simulink model "Mode_plus_Heading"  (R2015a)
settings: Solver=ode45  StartTime=0.0  StopTime=10.0  RelTol=1e-3
libraries: simulink x11, discretizing x1
settings Model: Creator=teme  LastModifiedBy=teme

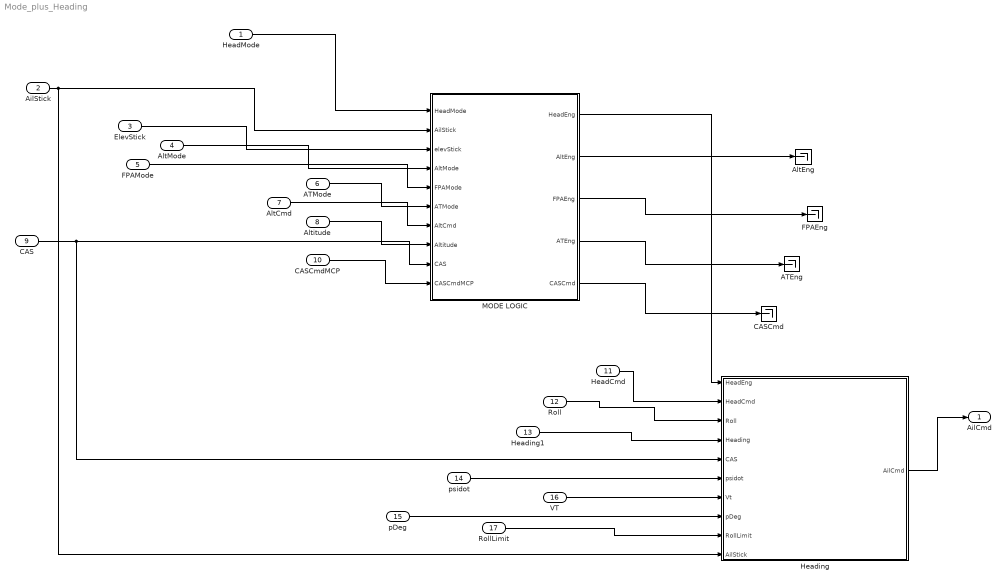
== system Mode_plus_Heading ==
  HeadMode : Inport
  AilStick : Inport  Port=2
  ElevStick : Inport  Port=3
  AltMode : Inport  Port=4
  FPAMode : Inport  Port=5
  ATMode : Inport  Port=6
  AltCmd : Inport  Port=7
  Altitude : Inport  Port=8
  CAS : Inport  Port=9
  CASCmdMCP : Inport  Port=10
  HeadCmd : Inport  Port=11
  "Roll " : Inport  Port=12
  Heading1 : Inport  Port=13
  psidot : Inport  Port=14
  pDeg : Inport  Port=15
  VT : Inport  Port=16
  RollLimit : Inport  Port=17
  ATEng : Terminator
  AltEng : Terminator
  CASCmd : Terminator
  FPAEng : Terminator
  Heading : Subsystem  TreatAsAtomicUnit=on
  MODE LOGIC : Subsystem  TreatAsAtomicUnit=on
  AilCmd : Outport
  wires:
  HeadMode/1 -> MODE LOGIC/1(HeadMode)
  AilStick/1 -> Heading/10(AilStick), MODE LOGIC/2(AilStick)
  AltMode/1 -> MODE LOGIC/4(AltMode)
  FPAMode/1 -> MODE LOGIC/5(FPAMode)
  ATMode/1 -> MODE LOGIC/6(ATMode)
  CASCmdMCP/1 -> MODE LOGIC/10(CASCmdMCP)
  MODE LOGIC/1(HeadEng) -> Heading/1(HeadEng)
  CAS/1 -> Heading/5(CAS), MODE LOGIC/9(CAS)
  AltCmd/1 -> MODE LOGIC/7(AltCmd)
  Altitude/1 -> MODE LOGIC/8(Altitude)
  ElevStick/1 -> MODE LOGIC/3(elevStick)
  Heading/1(AilCmd) -> AilCmd/1
  HeadCmd/1 -> Heading/2(HeadCmd)
  "Roll "/1 -> Heading/3(Roll)
  Heading1/1 -> Heading/4(Heading)
  psidot/1 -> Heading/6(psidot)
  pDeg/1 -> Heading/8(pDeg)
  VT/1 -> Heading/7(Vt)
  RollLimit/1 -> Heading/9(RollLimit)
  MODE LOGIC/2(AltEng) -> AltEng/1
  MODE LOGIC/3(FPAEng) -> FPAEng/1
  MODE LOGIC/4(ATEng) -> ATEng/1
  MODE LOGIC/5(CASCmd) -> CASCmd/1

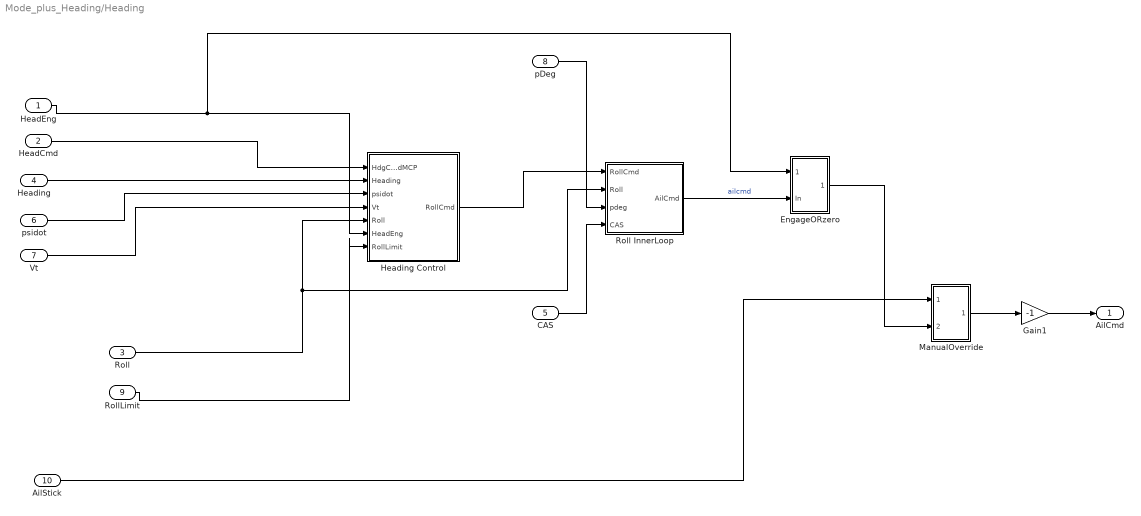
== system Mode_plus_Heading/Heading ==
  HeadEng : Inport
  HeadCmd : Inport  Port=2
  Roll : Inport  Port=3
  Heading : Inport  Port=4
  CAS : Inport  Port=5
  psidot : Inport  Port=6
  Vt : Inport  Port=7
  pDeg : Inport  Port=8
  RollLimit : Inport  Port=9
  AilStick : Inport  Port=10
  EngageORzero : Subsystem
  Gain1 : Gain  RequirementInfo={} %GIDa_6d55ac65_202a_4981_a4f5_213afcb30605  Gain=-1  SaturateOnIntegerOverflow=on  OutDataTypeStr=Inherit: Same as input  ParamDataTypeStr=Inherit: Same as input
  Heading Control : Subsystem  RequirementInfo={'other' '..\..\tcm_requirements.docx' '@Simulink_requirement_item_16' 'true' 'Heading Control' '' } %GIDa_029c738f_f50b_45d2_a289_cf2e96dbaa78  TreatAsAtomicUnit=on
  ManualOverride : Subsystem
  Roll InnerLoop : Subsystem  RequirementInfo={'other' '..\..\tcm_requirements.docx' '@Simulink_requirement_item_18' 'true' 'Roll InnerLoop' '' } %GIDa_cbfef998_9b02_4a35_a4cd_5451b3fb610d  TreatAsAtomicUnit=on
  AilCmd : Outport
  wires:
  pDeg/1 -> Roll InnerLoop/3(pdeg)
  Vt/1 -> Heading Control/4(Vt)
  psidot/1 -> Heading Control/3(psidot)
  Heading/1 -> Heading Control/2(Heading)
  Roll/1 -> Heading Control/5(Roll), Roll InnerLoop/2(Roll)
  Heading Control/1(RollCmd) -> Roll InnerLoop/1(RollCmd)
  Roll InnerLoop/1(AilCmd) -> EngageORzero/2(In)  "ailcmd"
  HeadCmd/1 -> Heading Control/1(HdgCmdMCP)
  HeadEng/1 -> EngageORzero/1(Engage), Heading Control/6(HeadEng)
  CAS/1 -> Roll InnerLoop/4(CAS)
  RollLimit/1 -> Heading Control/7(RollLimit)
  ManualOverride/1(Out) -> Gain1/1
  AilStick/1 -> ManualOverride/1(Man)
  Gain1/1 -> AilCmd/1
  EngageORzero/1(Out) -> ManualOverride/2(Auto)

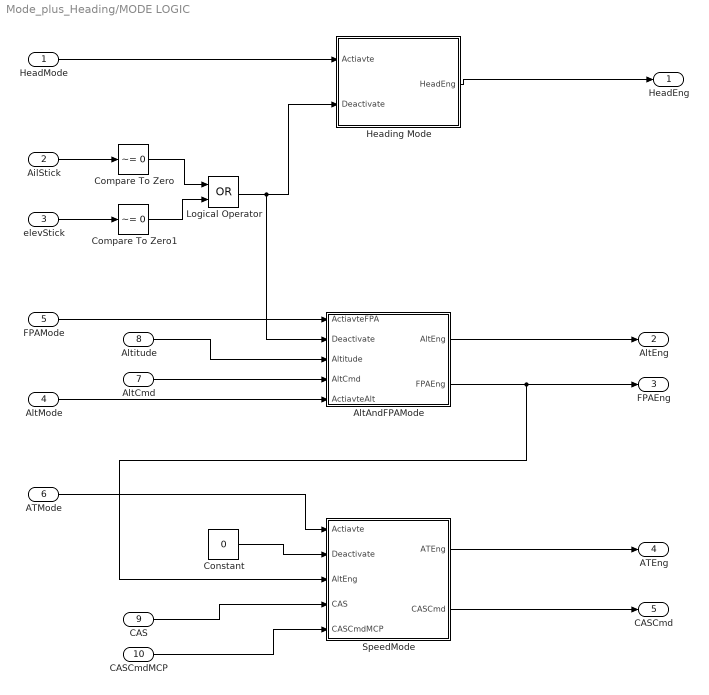
== system Mode_plus_Heading/MODE LOGIC ==
  HeadMode : Inport
  AilStick : Inport  Port=2
  elevStick : Inport  Port=3
  AltMode : Inport  Port=4
  FPAMode : Inport  Port=5
  ATMode : Inport  Port=6
  AltCmd : Inport  Port=7
  Altitude : Inport  Port=8
  CAS : Inport  Port=9
  CASCmdMCP : Inport  Port=10
  AltAndFPAMode : Subsystem  TreatAsAtomicUnit=on
  Compare To Zero : simulink/Logic and Bit Operations/Compare To Zero  relop=~=  OutDataTypeStr=boolean
  Compare To Zero1 : simulink/Logic and Bit Operations/Compare To Zero  relop=~=  OutDataTypeStr=boolean
  Constant : Constant  Value=0
  Heading Mode : Subsystem  TreatAsAtomicUnit=on
  Logical Operator : Logic  Operator=OR  AllPortsSameDT=off  OutDataTypeStr=boolean
  SpeedMode : Subsystem  TreatAsAtomicUnit=on
  HeadEng : Outport
  AltEng : Outport  Port=2
  FPAEng : Outport  Port=3
  ATEng : Outport  Port=4
  CASCmd : Outport  Port=5
  wires:
  SpeedMode/1(ATEng) -> ATEng/1
  AilStick/1 -> Compare To Zero/1
  Constant/1 -> SpeedMode/2(Deactivate)
  AltAndFPAMode/2(FPAEng) -> FPAEng/1, SpeedMode/3(AltEng)
  AltAndFPAMode/1(AltEng) -> AltEng/1
  Heading Mode/1(HeadEng) -> HeadEng/1
  HeadMode/1 -> Heading Mode/1(Actiavte)
  Compare To Zero1/1 -> Logical Operator/2
  Compare To Zero/1 -> Logical Operator/1
  elevStick/1 -> Compare To Zero1/1
  ATMode/1 -> SpeedMode/1(Actiavte)
  FPAMode/1 -> AltAndFPAMode/1(ActiavteFPA)
  Altitude/1 -> AltAndFPAMode/3(Altitude)
  AltMode/1 -> AltAndFPAMode/5(ActiavteAlt)
  Logical Operator/1 -> AltAndFPAMode/2(Deactivate), Heading Mode/2(Deactivate)
  CASCmdMCP/1 -> SpeedMode/5(CASCmdMCP)
  AltCmd/1 -> AltAndFPAMode/4(AltCmd)
  SpeedMode/2(CASCmd) -> CASCmd/1
  CAS/1 -> SpeedMode/4(CAS)

== system Mode_plus_Heading/Heading/EngageORzero ==
  Engage : Inport
  In : Inport  Port=2
  Logical Operator5 : Logic  RequirementInfo={} %GIDa_6b22acc9_652a_4444_ba60_66174211b3d7  AllPortsSameDT=off  OutDataTypeStr=boolean
  Switch1 : Switch  RequirementInfo={} %GIDa_a25acb75_51aa_42d7_a9cb_36d9cbb78c82  Threshold=0.5
  zero10 : Constant  RequirementInfo={} %GIDa_53b8c13b_6898_41e6_9738_617635f10221
  zero9 : Constant  RequirementInfo={} %GIDa_0f665773_e07d_469a_a003_01a4a005c292  Value=0
  Out : Outport
  wires:
  Engage/1 -> Logical Operator5/1
  zero10/1 -> Logical Operator5/2
  zero9/1 -> Switch1/3
  In/1 -> Switch1/1
  Logical Operator5/1 -> Switch1/2
  Switch1/1 -> Out/1

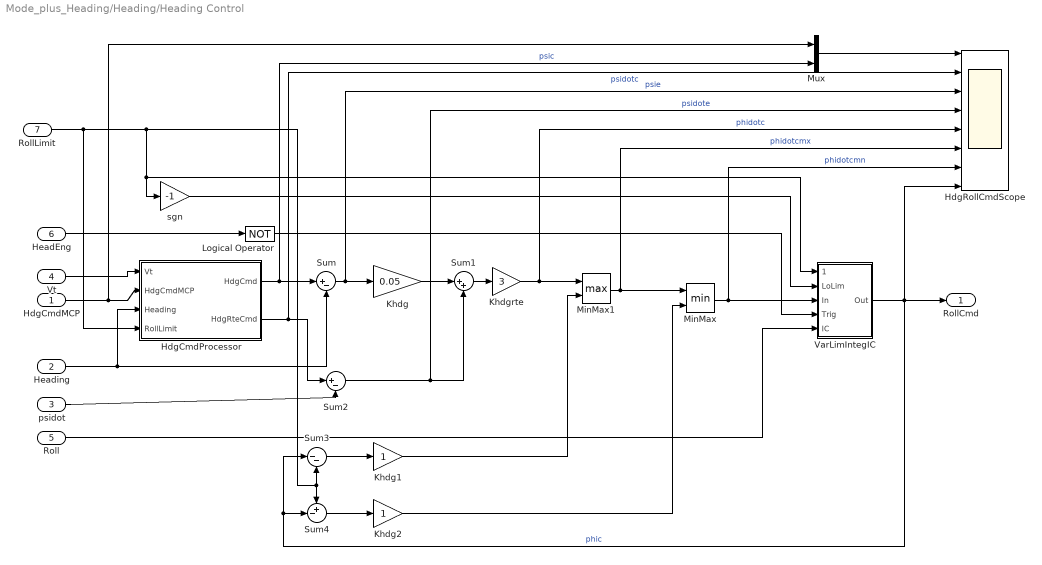
== system Mode_plus_Heading/Heading/Heading Control ==
  HdgCmdMCP : Inport  RequirementInfo={} %GIDa_1cca2c5c_8ee7_4499_91b8_56e2b6de226b
  Heading : Inport  RequirementInfo={} %GIDa_335b309e_b3fa_45a8_b4d1_17ef1ad18bf7  Port=2
  psidot : Inport  RequirementInfo={} %GIDa_0ad6fda9_8653_402a_9e5f_aea66e3ef369  Port=3
  Vt : Inport  RequirementInfo={} %GIDa_f5693dda_631a_4bfe_baea_8b34b02d8022  Port=4
  Roll : Inport  RequirementInfo={} %GIDa_593befd8_2743_476a_a356_0063a557a98d  Port=5
  HeadEng : Inport  RequirementInfo={} %GIDa_e8b59cf9_df4b_4ada_848e_4da61a3fd8b6  Port=6
  RollLimit : Inport  Port=7
  HdgCmdProcessor : Subsystem  RequirementInfo={} %GIDa_26e06564_c060_46ec_be4a_5847d57d6a81
  HdgRollCmdScope : Scope  NumInputPorts=8
      settings: RequirementInfo={} %GIDa_862353d9_0e7c_4d5b_85e1_9c9746c3fb38  YMin=-30~-30~-10~-10~-4~-10~0~-5  YMax=30~30~10~10~4~10~1~5  SaveName=ScopeData7
  Khdg : Gain  RequirementInfo={} %GIDa_c081e4bf_f383_4484_b7bd_3abc2cab8bec  Gain=0.05
  Khdg1 : Gain  RequirementInfo={} %GIDa_08836d3b_c1d7_4517_b088_b37e47d972bd
  Khdg2 : Gain  RequirementInfo={} %GIDa_3aec3149_958f_47ac_94ee_3d28a77fc3f5
  Khdgrte : Gain  RequirementInfo={} %GIDa_53d347bb_462f_4886_bdb2_badb643f02f4  Gain=3
  Logical Operator : Logic  RequirementInfo={} %GIDa_4b58cabb_2297_487d_8b60_ff4175741a78  Operator=NOT  AllPortsSameDT=off  OutDataTypeStr=boolean
  MinMax : MinMax  RequirementInfo={} %GIDa_e41d7ecf_e4e1_4710_b8b1_1fc040f0e9f7  Inputs=2
  MinMax1 : MinMax  RequirementInfo={} %GIDa_a4542adf_d925_494d_a294_9fe772a2ae1b  Function=max  Inputs=2
  Mux : Mux  RequirementInfo={} %GIDa_470c3405_5717_4020_8437_1a783ba94da4  Inputs=2
  Sum : Sum  RequirementInfo={} %GIDa_6c1efd1c_9252_4e5c_91dd_39c700892261  Inputs=|+-
  Sum1 : Sum  RequirementInfo={} %GIDa_6cd8dae3_1c4e_4eaf_8404_21dd295850e0  Inputs=|++
  Sum2 : Sum  RequirementInfo={} %GIDa_9d15b97d_5642_4675_a5ca_204c66429b4e  Inputs=|+-
  Sum3 : Sum  RequirementInfo={} %GIDa_2fe000b9_a62e_4a0f_869a_3cd4af55113b  Inputs=|--
  Sum4 : Sum  RequirementInfo={} %GIDa_c46e2e29_3542_4ab2_a31d_585bcdcc8614  Inputs=+-|
  VarLimIntegIC : Subsystem  RequirementInfo={} %GIDa_71edeeee_c821_4f10_9933_03fc141b3c8d
  sgn : Gain  RequirementInfo={} %GIDa_f2aeabed_4671_4607_b0d8_c27b93e0bf37  Gain=-1
  RollCmd : Outport  RequirementInfo={} %GIDa_4ce52d3c_e4b9_4db6_a642_099518279411
  wires:
  Heading/1 -> Sum/2, HdgCmdProcessor/3(Heading)
  HdgCmdProcessor/1(HdgCmd) -> Sum/1, Mux/2  "psic"
  Sum/1 -> Khdg/1, HdgRollCmdScope/3  "psie"
  Khdg/1 -> Sum1/1
  Sum2/1 -> Sum1/2, HdgRollCmdScope/4  "psidote"
  HdgCmdProcessor/2(HdgRteCmd) -> Sum2/1, HdgRollCmdScope/2  "psidotc"
  psidot/1 -> Sum2/2
  Vt/1 -> HdgCmdProcessor/1(Vt)
  HdgCmdMCP/1 -> HdgCmdProcessor/2(HdgCmdMCP), Mux/1
  VarLimIntegIC/1(Out) -> RollCmd/1, Sum3/1, Sum4/2, HdgRollCmdScope/8  "phic"
  RollLimit/1 -> HdgCmdProcessor/4(RollLimit), Sum4/1, Sum3/2, VarLimIntegIC/1(UpLim), sgn/1
  sgn/1 -> VarLimIntegIC/2(LoLim)
  Sum1/1 -> Khdgrte/1
  MinMax1/1 -> MinMax/1, HdgRollCmdScope/6  "phidotcmx"
  MinMax/1 -> VarLimIntegIC/3(In), HdgRollCmdScope/7  "phidotcmn"
  HeadEng/1 -> Logical Operator/1
  Sum3/1 -> Khdg1/1
  Sum4/1 -> Khdg2/1
  Khdg1/1 -> MinMax1/2
  Khdg2/1 -> MinMax/2
  Roll/1 -> VarLimIntegIC/5(IC)
  Khdgrte/1 -> MinMax1/1, HdgRollCmdScope/5  "phidotc"
  Logical Operator/1 -> VarLimIntegIC/4(Trig)
  Mux/1 -> HdgRollCmdScope/1

== system Mode_plus_Heading/Heading/ManualOverride ==
  Man : Inport
  Auto : Inport  Port=2
  Switch1 : Switch  RequirementInfo={} %GIDa_e9c946ef_c3db_4bff_aed9_ae767ef4d81f  Criteria=u2 ~= 0  Threshold=0.5
  Out : Outport
  wires:
  Man/1 -> Switch1/3, Switch1/2
  Auto/1 -> Switch1/1
  Switch1/1 -> Out/1

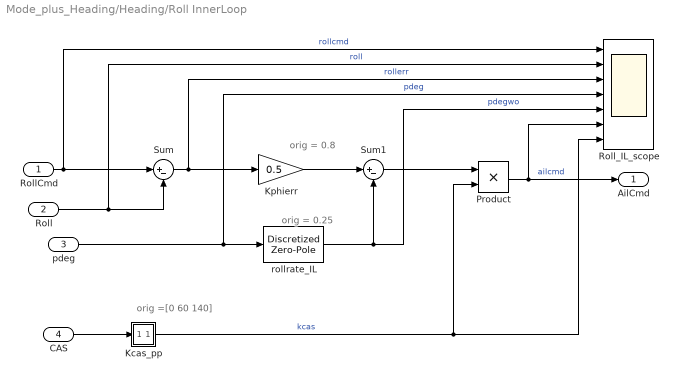
== system Mode_plus_Heading/Heading/Roll InnerLoop ==
  note: orig =[0 60 140]
  note: orig = 0.25
  note: orig = 0.8
  RollCmd : Inport  RequirementInfo={} %GIDa_d025a660_cca0_4be3_be06_f9a4dfc86269
  Roll : Inport  RequirementInfo={} %GIDa_e417ba20_aa70_4b95_9916_e8dd209e2685  Port=2
  pdeg : Inport  RequirementInfo={} %GIDa_36f75b87_1287_4d91_9dd1_6a1f7713c617  Port=3
  CAS : Inport  RequirementInfo={} %GIDa_f5e5b1c2_d48b_4547_abd4_42af90480919  Port=4
  Kcas_pp : Subsystem  TreatAsAtomicUnit=on
  Kphierr : Gain  RequirementInfo={} %GIDa_4a49e338_8293_4eab_bd1b_6b3b87e03ed9  Gain=0.5
  Product : Product  RequirementInfo={} %GIDa_b6bb309d_f019_4adc_b849_d0e1434187e8  RndMeth=Zero
  Roll_IL_scope : Scope  NumInputPorts=7
      settings: RequirementInfo={} %GIDa_cdfba529_0977_4006_adbd_37c3f846a021  YMin=-30~-30~-10~-10~-4~-10~0  YMax=30~30~10~10~4~10~1  SaveName=ScopeData5
  Sum : Sum  RequirementInfo={} %GIDa_8570fcab_2296_4031_bbbc_4321a9111662  Inputs=|+-
  Sum1 : Sum  RequirementInfo={} %GIDa_b2216589_c422_4707_aad7_b64095d3debb  Inputs=|+-
  rollrate_IL : discretizing/Discretized Zero-Pole  RequirementInfo={} %GIDa_636569be_bc7e_4244_84a4_4a62b7fc0808  Zeros=0  Poles=-0.5  Gain=0.00645  AbsTol=auto  SampleTime=1.0  method=zoh  Wc=1
  AilCmd : Outport  RequirementInfo={} %GIDa_5926b7f8_9769_4f97_a0ed_432ffd436784
  wires:
  Product/1 -> AilCmd/1, Roll_IL_scope/6  "ailcmd"
  Kcas_pp/1(Out) -> Product/2, Roll_IL_scope/7  "kcas"
  Sum1/1 -> Product/1
  CAS/1 -> Kcas_pp/1(In)
  rollrate_IL/1 -> Sum1/2, Roll_IL_scope/5  "pdegwo"
  pdeg/1 -> rollrate_IL/1, Roll_IL_scope/4  "pdeg"
  Kphierr/1 -> Sum1/1
  Roll/1 -> Sum/2, Roll_IL_scope/2  "roll"
  Sum/1 -> Kphierr/1, Roll_IL_scope/3  "rollerr"
  RollCmd/1 -> Sum/1, Roll_IL_scope/1  "rollcmd"

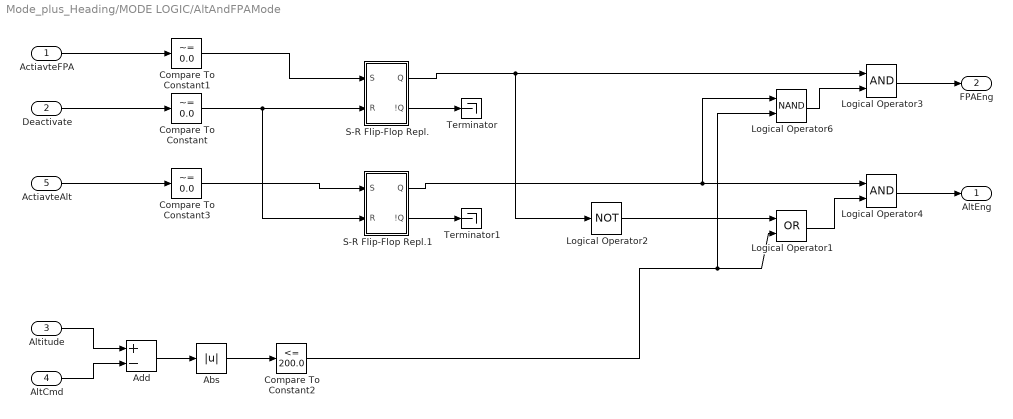
== system Mode_plus_Heading/MODE LOGIC/AltAndFPAMode ==
  ActiavteFPA : Inport
  Deactivate : Inport  Port=2
  Altitude : Inport  Port=3
  AltCmd : Inport  Port=4
  ActiavteAlt : Inport  Port=5
  Abs : Abs
  Add : Sum  Inputs=+-
  Compare To Constant : simulink/Logic and Bit Operations/Compare To Constant  relop=~=  const=0.0  OutDataTypeStr=boolean
  Compare To Constant1 : simulink/Logic and Bit Operations/Compare To Constant  relop=~=  const=0.0  OutDataTypeStr=boolean
  Compare To Constant2 : simulink/Logic and Bit Operations/Compare To Constant  relop=<=  const=200.0  OutDataTypeStr=boolean
  Compare To Constant3 : simulink/Logic and Bit Operations/Compare To Constant  relop=~=  const=0.0  OutDataTypeStr=boolean
  Logical Operator1 : Logic  Operator=OR  AllPortsSameDT=off  OutDataTypeStr=boolean
  Logical Operator2 : Logic  Operator=NOT  AllPortsSameDT=off  OutDataTypeStr=boolean
  Logical Operator3 : Logic  AllPortsSameDT=off  OutDataTypeStr=boolean
  Logical Operator4 : Logic  AllPortsSameDT=off  OutDataTypeStr=boolean
  Logical Operator6 : Logic  Operator=NAND  AllPortsSameDT=off  OutDataTypeStr=boolean
  S-R Flip-Flop Repl. : Subsystem
  S-R Flip-Flop Repl.1 : Subsystem
  Terminator : Terminator
  Terminator1 : Terminator
  AltEng : Outport
  FPAEng : Outport  Port=2
  wires:
  S-R Flip-Flop Repl./2(!Q) -> Terminator/1
  ActiavteFPA/1 -> Compare To Constant1/1
  S-R Flip-Flop Repl./1(Q) -> Logical Operator3/1, Logical Operator2/1
  Deactivate/1 -> Compare To Constant/1
  Compare To Constant1/1 -> S-R Flip-Flop Repl./1(S)
  S-R Flip-Flop Repl.1/2(!Q) -> Terminator1/1
  S-R Flip-Flop Repl.1/1(Q) -> Logical Operator6/1, Logical Operator4/1
  Compare To Constant3/1 -> S-R Flip-Flop Repl.1/1(S)
  Compare To Constant/1 -> S-R Flip-Flop Repl.1/2(R), S-R Flip-Flop Repl./2(R)
  ActiavteAlt/1 -> Compare To Constant3/1
  Altitude/1 -> Add/1
  AltCmd/1 -> Add/2
  Add/1 -> Abs/1
  Abs/1 -> Compare To Constant2/1
  Logical Operator3/1 -> FPAEng/1
  Logical Operator2/1 -> Logical Operator1/1
  Logical Operator4/1 -> AltEng/1
  Compare To Constant2/1 -> Logical Operator6/2, Logical Operator1/2
  Logical Operator1/1 -> Logical Operator4/2
  Logical Operator6/1 -> Logical Operator3/2

== system Mode_plus_Heading/MODE LOGIC/Heading Mode ==
  Actiavte : Inport
  Deactivate : Inport  Port=2
  Compare To Constant : simulink/Logic and Bit Operations/Compare To Constant  relop=~=  const=0.0  OutDataTypeStr=boolean
  Compare To Constant1 : simulink/Logic and Bit Operations/Compare To Constant  relop=~=  const=0.0  OutDataTypeStr=boolean
  S-R Flip-Flop Repl. : Subsystem
  Terminator : Terminator
  HeadEng : Outport
  wires:
  S-R Flip-Flop Repl./2(!Q) -> Terminator/1
  Actiavte/1 -> Compare To Constant1/1
  S-R Flip-Flop Repl./1(Q) -> HeadEng/1
  Deactivate/1 -> Compare To Constant/1
  Compare To Constant1/1 -> S-R Flip-Flop Repl./1(S)
  Compare To Constant/1 -> S-R Flip-Flop Repl./2(R)

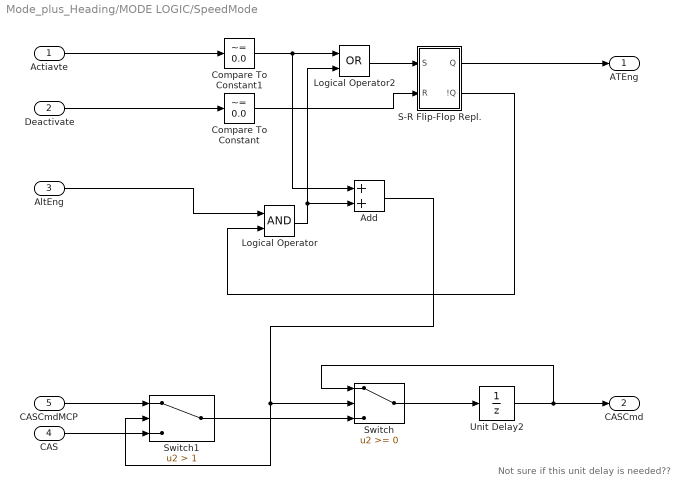
== system Mode_plus_Heading/MODE LOGIC/SpeedMode ==
  note: Not sure if this unit delay is needed??
  Actiavte : Inport
  Deactivate : Inport  Port=2
  AltEng : Inport  Port=3
  CAS : Inport  Port=4
  CASCmdMCP : Inport  Port=5
  Add : Sum
  Compare To Constant : simulink/Logic and Bit Operations/Compare To Constant  relop=~=  const=0.0  OutDataTypeStr=boolean
  Compare To Constant1 : simulink/Logic and Bit Operations/Compare To Constant  relop=~=  const=0.0  OutDataTypeStr=boolean
  Logical Operator : Logic  AllPortsSameDT=off  OutDataTypeStr=boolean
  Logical Operator2 : Logic  Operator=OR  AllPortsSameDT=off  OutDataTypeStr=boolean
  S-R Flip-Flop Repl. : Subsystem
  Switch : Switch
  Switch1 : Switch  Criteria=u2 > Threshold  Threshold=1
  Unit Delay2 : UnitDelay  SampleTime=-1
  ATEng : Outport
  CASCmd : Outport  Port=2
  wires:
  Actiavte/1 -> Compare To Constant1/1
  S-R Flip-Flop Repl./1(Q) -> ATEng/1
  Deactivate/1 -> Compare To Constant/1
  Compare To Constant/1 -> S-R Flip-Flop Repl./2(R)
  AltEng/1 -> Logical Operator/1
  Logical Operator2/1 -> S-R Flip-Flop Repl./1(S)
  Logical Operator/1 -> Add/2, Logical Operator2/2
  CAS/1 -> Switch1/3
  CASCmdMCP/1 -> Switch1/1
  Compare To Constant1/1 -> Add/1, Logical Operator2/1
  Add/1 -> Switch1/2, Switch/2
  Switch1/1 -> Switch/3
  Switch/1 -> Unit Delay2/1
  Unit Delay2/1 -> Switch/1, CASCmd/1
  S-R Flip-Flop Repl./2(!Q) -> Logical Operator/2

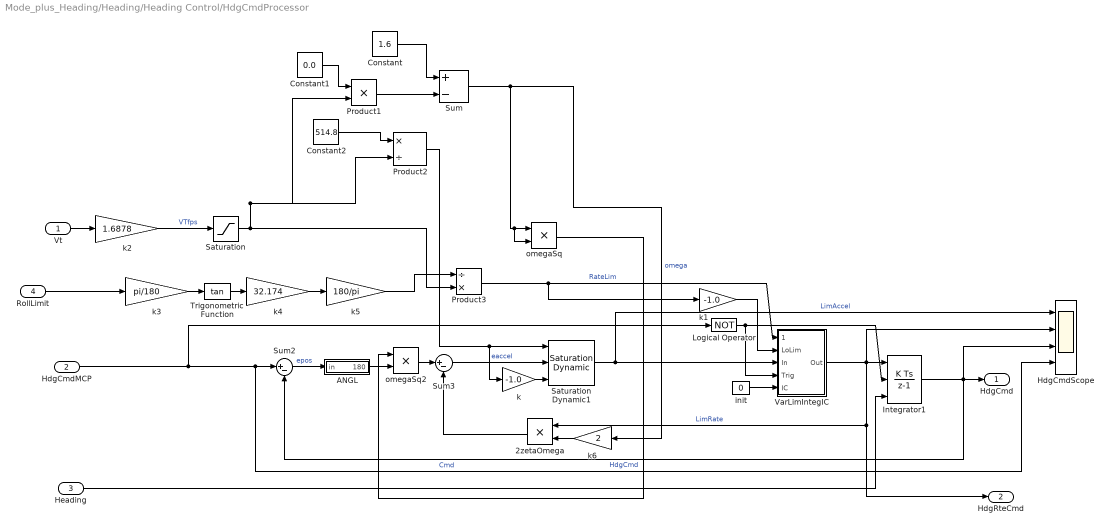
== system Mode_plus_Heading/Heading/Heading Control/HdgCmdProcessor ==
  Vt : Inport  RequirementInfo={} %GIDa_466651cd_7f6b_413f_959c_d2f22fb33a11
  HdgCmdMCP : Inport  RequirementInfo={} %GIDa_ae519e0f_0fd0_4cbd_b8f6_352ace01c202  Port=2
  Heading : Inport  RequirementInfo={} %GIDa_acc7b106_bfa8_4c68_a4ce_753e4271b39e  Port=3
  RollLimit : Inport  Port=4
  2zetaOmega : Product  RequirementInfo={} %GIDa_bd0f0ab9_3df7_4288_bc18_2f6d8104ad8c  RndMeth=Zero
  ANGL : Subsystem  RequirementInfo={} %GIDa_5f0af73c_00da_4b95_896f_21709d1258bb
  Constant : Constant  Value=1.6
  Constant1 : Constant  Value=0.0
  Constant2 : Constant  Value=514.8
  HdgCmdScope : Scope  NumInputPorts=4
      settings: RequirementInfo={} %GIDa_6a29be8f_c2d6_453a_bef2_65f6038f4f3f  YMin=-2~-4~-40~-40  YMax=2~4~40~40  SaveName=ScopeData6
  Integrator1 : DiscreteIntegrator  ExternalReset=level  InitialConditionSource=external  SampleTime=1.0  mask(DiscretizedDiscreteIntegrator){}
      mask init:
      | %zoh
  Logical Operator : Logic  RequirementInfo={} %GIDa_91b56384_6bc5_48f7_99d5_59c3b87c3ce7  Operator=NOT  AllPortsSameDT=off  OutDataTypeStr=boolean
  Product1 : Product  RndMeth=Zero
  Product2 : Product  Inputs=*/  RndMeth=Zero
  Product3 : Product  Inputs=/*  RndMeth=Zero
  Saturation : Saturate  RequirementInfo={} %GIDa_d0b25274_da4b_4ee3_b878_fc1af8ef952a  UpperLimit=1000  LowerLimit=0.0001
  Saturation Dynamic1 : simulink/Discontinuities/Saturation Dynamic  RequirementInfo={} %GIDa_3c1bb0e4_035b_467b_b908_73d0679fa8c4  OutMin=[]  OutMax=[]  OutDataTypeStr=Inherit: Same as second input  OutDataType=fixdt(1, 16)  OutScaling=2^-10  DoSatur=off
  Sum : Sum  Inputs=+-
  Sum2 : Sum  RequirementInfo={} %GIDa_838fdc30_721d_4f05_b4bd_39ad69dce7db  Inputs=|+-
  Sum3 : Sum  RequirementInfo={} %GIDa_add2bfe6_01b5_48a9_a979_92289a564191  Inputs=|+-
  Trigonometric Function : Trigonometry  RequirementInfo={} %GIDa_6ee22cce_8025_4b18_aafe_7b752fcee01b  Operator=tan
  VarLimIntegIC : Subsystem  RequirementInfo={} %GIDa_1079489d_11fe_487a_a9b6_1afe68a2d042
  init : Constant  RequirementInfo={} %GIDa_7d2a4e74_a111_4116_8bd2_0ad66af5b0b8  Value=0
  k : Gain  RequirementInfo={} %GIDa_217db761_d5da_44b3_b86d_50f3808c63df  Gain=-1.0
  k1 : Gain  RequirementInfo={} %GIDa_c738a275_db1d_49e7_8241_29f9dc740d55  Gain=-1.0
  k2 : Gain  RequirementInfo={} %GIDa_e1c70c52_d5bd_4847_bba2_580db545f9e7  Gain=1.6878
  k3 : Gain  RequirementInfo={} %GIDa_90e5bea6_e9d6_4de2_9e7c_568b40e8935d  Gain=pi/180
  k4 : Gain  RequirementInfo={} %GIDa_c95271b7_f922_40b3_a20f_3ff986d2bf93  Gain=32.174
  k5 : Gain  RequirementInfo={} %GIDa_62d5d32d_48dc_4e00_95de_a9f551b1c6a3  Gain=180/pi
  k6 : Gain  RequirementInfo={} %GIDa_74395756_a11d_4c0b_95f6_b640da60b068  Gain=2
  omegaSq : Product  RequirementInfo={} %GIDa_f7d3aa6b_daca_4a13_b172_f703fc474f5e  RndMeth=Zero
  omegaSq2 : Product  RequirementInfo={} %GIDa_3e8c5e93_e091_404a_9a70_e69aeb24bdb6  RndMeth=Zero
  HdgCmd : Outport  RequirementInfo={} %GIDa_4e47a000_0398_4458_9a88_cb69c0c50bdd
  HdgRteCmd : Outport  RequirementInfo={} %GIDa_54d54c5f_9642_4dfe_b6f2_8b7e6f9e9a5a  Port=2
  wires:
  Integrator1/1 -> Sum2/2, HdgCmd/1, HdgCmdScope/3  "HdgCmd"
  Vt/1 -> k2/1
  k2/1 -> Saturation/1  "VTfps"
  k/1 -> Saturation Dynamic1/3
  RollLimit/1 -> k3/1
  Sum3/1 -> Saturation Dynamic1/2  "eaccel"
  Saturation Dynamic1/1 -> VarLimIntegIC/3(In), HdgCmdScope/1  "LimAccel"
  k3/1 -> Trigonometric Function/1
  Trigonometric Function/1 -> k4/1
  k4/1 -> k5/1
  k5/1 -> Product3/1
  Product3/1 -> VarLimIntegIC/1(UpLim), k1/1  "RateLim"
  k1/1 -> VarLimIntegIC/2(LoLim)
  VarLimIntegIC/1(Out) -> Integrator1/1, HdgCmdScope/2, 2zetaOmega/1, HdgRteCmd/1  "LimRate"
  k6/1 -> 2zetaOmega/2
  2zetaOmega/1 -> Sum3/2
  init/1 -> VarLimIntegIC/5(IC)
  omegaSq/1 -> omegaSq2/1
  omegaSq2/1 -> Sum3/1
  Sum2/1 -> ANGL/1(in)  "epos"
  HdgCmdMCP/1 -> Logical Operator/1, Sum2/1, HdgCmdScope/4  "Cmd"
  ANGL/1(180) -> omegaSq2/2
  Logical Operator/1 -> VarLimIntegIC/4(Trig), Integrator1/2
  Saturation/1 -> Product1/2, Product2/2, Product3/2
  Heading/1 -> Integrator1/3
  Product2/1 -> Saturation Dynamic1/1, k/1
  Constant/1 -> Sum/1
  Constant1/1 -> Product1/1
  Product1/1 -> Sum/2
  Constant2/1 -> Product2/1
  Sum/1 -> k6/1, omegaSq/1, omegaSq/2  "omega"

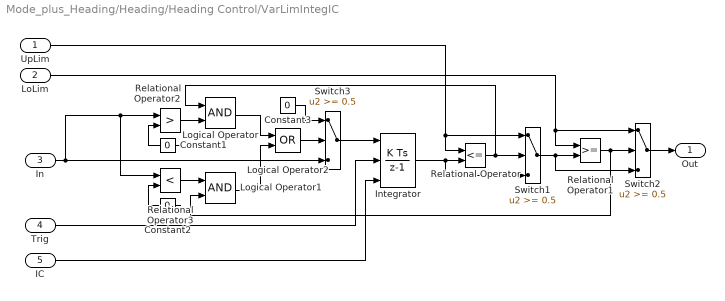
== system Mode_plus_Heading/Heading/Heading Control/VarLimIntegIC ==
  UpLim : Inport  RequirementInfo={} %GIDa_0778c5f4_39de_4b0c_991c_83089b08ca8a
  LoLim : Inport  RequirementInfo={} %GIDa_448fa833_a29e_45fb_80f3_326b2c64b719  Port=2
  In : Inport  RequirementInfo={} %GIDa_d3ef3527_b6e3_461a_8708_0529431b64dc  Port=3
  Trig : Inport  RequirementInfo={} %GIDa_6ebe9539_e2a6_41f3_aedd_40ba92f31e5e  Port=4
  IC : Inport  RequirementInfo={} %GIDa_e1ebf0cf_42b8_4c18_8595_be81bac9db69  Port=5
  Constant1 : Constant  RequirementInfo={} %GIDa_75e7403a_dfcf_4330_9fa8_27225d4b12fc  Value=0
  Constant2 : Constant  RequirementInfo={} %GIDa_3951a41b_a413_48e6_8e04_86cf93f585e7  Value=0
  Constant3 : Constant  RequirementInfo={} %GIDa_44ac0f43_b5aa_4afc_b424_50d763880c36  Value=0
  Integrator : DiscreteIntegrator  ExternalReset=level  InitialConditionSource=external  SampleTime=1.0  mask(DiscretizedDiscreteIntegrator){}
      mask init:
      | %zoh
  Logical Operator : Logic  RequirementInfo={} %GIDa_9eb0ae12_a2eb_47a0_817d_b37632c93507  AllPortsSameDT=off
  Logical Operator1 : Logic  RequirementInfo={} %GIDa_ba6a9ad9_4185_4eeb_a553_c67232b44ead  AllPortsSameDT=off
  Logical Operator2 : Logic  RequirementInfo={} %GIDa_7814430c_a53b_4fd8_9b9b_4b0f33b90b31  Operator=OR  AllPortsSameDT=off
  Relational Operator : RelationalOperator  RequirementInfo={} %GIDa_ed30788a_60fb_4430_8f42_bc98339f4005  Operator=<=
  Relational Operator1 : RelationalOperator  RequirementInfo={} %GIDa_8d8301bc_fc54_428d_9b8d_1dc8c181918b
  Relational Operator2 : RelationalOperator  RequirementInfo={} %GIDa_3c178929_7d83_4b49_bf88_dbd29ed7fa35  Operator=>
  Relational Operator3 : RelationalOperator  RequirementInfo={} %GIDa_2e8bdf20_e6c2_4e45_b3d8_4669e6a8fbda  Operator=<
  Switch1 : Switch  RequirementInfo={} %GIDa_f0f767ce_ceda_4473_bc41_daa5516eb17a  Threshold=0.5  SaturateOnIntegerOverflow=on  InputSameDT=on
  Switch2 : Switch  RequirementInfo={} %GIDa_bc180920_7ceb_4401_b52f_14e8f0683ea5  Threshold=0.5  SaturateOnIntegerOverflow=on  InputSameDT=on
  Switch3 : Switch  RequirementInfo={} %GIDa_4f7c693a_ed1a_4c07_b68d_f024ed9afaed  Threshold=0.5  SaturateOnIntegerOverflow=on  InputSameDT=on
  Out : Outport  RequirementInfo={} %GIDa_fd631654_d2e3_4589_8acd_101e79f81c16
  wires:
  Relational Operator1/1 -> Logical Operator1/2, Switch2/2
  Switch1/1 -> Switch2/3, Relational Operator1/2
  LoLim/1 -> Relational Operator1/1, Switch2/1
  IC/1 -> Integrator/3
  Trig/1 -> Integrator/2
  Constant2/1 -> Relational Operator3/2
  Relational Operator3/1 -> Logical Operator1/1
  Logical Operator1/1 -> Logical Operator2/2
  Logical Operator/1 -> Logical Operator2/1
  Logical Operator2/1 -> Switch3/2
  Relational Operator2/1 -> Logical Operator/2
  Constant1/1 -> Relational Operator2/2
  In/1 -> Switch3/3, Relational Operator3/1, Relational Operator2/1
  Constant3/1 -> Switch3/1
  Switch3/1 -> Integrator/1
  Relational Operator/1 -> Logical Operator/1, Switch1/2
  Switch2/1 -> Out/1
  UpLim/1 -> Switch1/1, Relational Operator/1
  Integrator/1 -> Relational Operator/2, Switch1/3

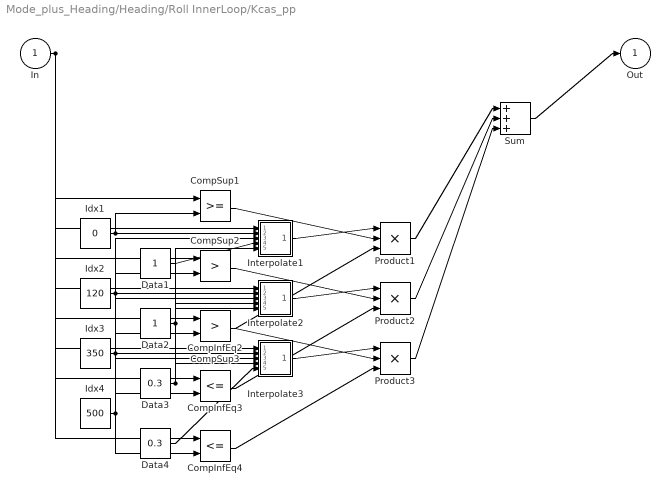
== system Mode_plus_Heading/Heading/Roll InnerLoop/Kcas_pp ==
  In : Inport
  CompInfEq2 : RelationalOperator  Operator=<=  InputSameDT=on
  CompInfEq3 : RelationalOperator  Operator=<=  InputSameDT=on
  CompInfEq4 : RelationalOperator  Operator=<=  InputSameDT=on
  CompSup1 : RelationalOperator  InputSameDT=on
  CompSup2 : RelationalOperator  Operator=>  InputSameDT=on
  CompSup3 : RelationalOperator  Operator=>  InputSameDT=on
  Data1 : Constant
  Data2 : Constant
  Data3 : Constant  Value=0.3
  Data4 : Constant  Value=0.3
  Idx1 : Constant  Value=0
  Idx2 : Constant  Value=120
  Idx3 : Constant  Value=350
  Idx4 : Constant  Value=500
  Interpolate1 : Subsystem
  Interpolate2 : Subsystem
  Interpolate3 : Subsystem
  Product1 : Product  Inputs=***  SaturateOnIntegerOverflow=on  RndMeth=Zero  OutDataTypeStr=Inherit: Same as first input
  Product2 : Product  Inputs=***  SaturateOnIntegerOverflow=on  RndMeth=Zero  OutDataTypeStr=Inherit: Same as first input
  Product3 : Product  Inputs=***  SaturateOnIntegerOverflow=on  RndMeth=Zero  OutDataTypeStr=Inherit: Same as first input
  Sum : Sum  Inputs=+++  SaturateOnIntegerOverflow=on  InputSameDT=on  OutDataTypeStr=Inherit: Same as first input
  Out : Outport
  wires:
  In/1 -> Interpolate1/1(InportIn), CompSup1/1, Interpolate2/1(InportIn), CompSup2/1, CompInfEq2/1, Interpolate3/1(InportIn), CompSup3/1, CompInfEq3/1, CompInfEq4/1
  Idx1/1 -> Interpolate1/2(InportIdx1), CompSup1/2
  Data1/1 -> Interpolate1/4(InportData1)
  Interpolate1/1(Out) -> Product1/1
  CompSup1/1 -> Product1/2
  CompInfEq2/1 -> Product1/3
  Product1/1 -> Sum/1
  Idx2/1 -> Interpolate2/2(InportIdx1), CompSup2/2, Interpolate1/3(InportIdx2), CompInfEq2/2
  Data2/1 -> Interpolate2/4(InportData1), Interpolate1/5(InportData2)
  Interpolate2/1(Out) -> Product2/1
  CompSup2/1 -> Product2/2
  CompInfEq3/1 -> Product2/3
  Product2/1 -> Sum/2
  Idx3/1 -> Interpolate3/2(InportIdx1), CompSup3/2, Interpolate2/3(InportIdx2), CompInfEq3/2
  Data3/1 -> Interpolate3/4(InportData1), Interpolate2/5(InportData2)
  Interpolate3/1(Out) -> Product3/1
  CompSup3/1 -> Product3/2
  CompInfEq4/1 -> Product3/3
  Product3/1 -> Sum/3
  Idx4/1 -> Interpolate3/3(InportIdx2), CompInfEq4/2
  Data4/1 -> Interpolate3/5(InportData2)
  Sum/1 -> Out/1

== system Mode_plus_Heading/MODE LOGIC/AltAndFPAMode/S-R Flip-Flop Repl. ==
  S : Inport
  R : Inport  Port=2
  Logical Operator : Logic  Operator=NAND  AllPortsSameDT=off  OutDataTypeStr=boolean
  Logical Operator1 : Logic  Operator=NAND  AllPortsSameDT=off  OutDataTypeStr=boolean
  Logical Operator2 : Logic  Operator=NOT  AllPortsSameDT=off  OutDataTypeStr=boolean
  Logical Operator3 : Logic  Operator=NOT  AllPortsSameDT=off  OutDataTypeStr=boolean
  Unit Delay : UnitDelay  SampleTime=-1
  Unit Delay1 : UnitDelay  InitialCondition=1  SampleTime=-1
  Q : Outport
  !Q : Outport  Port=2
  wires:
  Logical Operator/1 -> Unit Delay1/1, !Q/1
  Logical Operator1/1 -> Unit Delay/1, Q/1
  Unit Delay/1 -> Logical Operator/1
  Unit Delay1/1 -> Logical Operator1/2
  Logical Operator2/1 -> Logical Operator1/1
  Logical Operator3/1 -> Logical Operator/2
  R/1 -> Logical Operator3/1
  S/1 -> Logical Operator2/1

== system Mode_plus_Heading/MODE LOGIC/AltAndFPAMode/S-R Flip-Flop Repl.1 ==
  S : Inport
  R : Inport  Port=2
  Logical Operator : Logic  Operator=NAND  AllPortsSameDT=off  OutDataTypeStr=boolean
  Logical Operator1 : Logic  Operator=NAND  AllPortsSameDT=off  OutDataTypeStr=boolean
  Logical Operator2 : Logic  Operator=NOT  AllPortsSameDT=off  OutDataTypeStr=boolean
  Logical Operator3 : Logic  Operator=NOT  AllPortsSameDT=off  OutDataTypeStr=boolean
  Unit Delay : UnitDelay  SampleTime=-1
  Unit Delay1 : UnitDelay  InitialCondition=1  SampleTime=-1
  Q : Outport
  !Q : Outport  Port=2
  wires:
  Logical Operator/1 -> Unit Delay1/1, !Q/1
  Logical Operator1/1 -> Unit Delay/1, Q/1
  Unit Delay/1 -> Logical Operator/1
  Unit Delay1/1 -> Logical Operator1/2
  Logical Operator2/1 -> Logical Operator1/1
  Logical Operator3/1 -> Logical Operator/2
  R/1 -> Logical Operator3/1
  S/1 -> Logical Operator2/1

== system Mode_plus_Heading/MODE LOGIC/Heading Mode/S-R Flip-Flop Repl. ==
  S : Inport
  R : Inport  Port=2
  Logical Operator : Logic  Operator=NAND  AllPortsSameDT=off  OutDataTypeStr=boolean
  Logical Operator1 : Logic  Operator=NAND  AllPortsSameDT=off  OutDataTypeStr=boolean
  Logical Operator2 : Logic  Operator=NOT  AllPortsSameDT=off  OutDataTypeStr=boolean
  Logical Operator3 : Logic  Operator=NOT  AllPortsSameDT=off  OutDataTypeStr=boolean
  Unit Delay : UnitDelay  SampleTime=-1
  Unit Delay1 : UnitDelay  InitialCondition=1  SampleTime=-1
  Q : Outport
  !Q : Outport  Port=2
  wires:
  Logical Operator/1 -> Unit Delay1/1, !Q/1
  Logical Operator1/1 -> Unit Delay/1, Q/1
  Unit Delay/1 -> Logical Operator/1
  Unit Delay1/1 -> Logical Operator1/2
  Logical Operator2/1 -> Logical Operator1/1
  Logical Operator3/1 -> Logical Operator/2
  R/1 -> Logical Operator3/1
  S/1 -> Logical Operator2/1

== system Mode_plus_Heading/MODE LOGIC/SpeedMode/S-R Flip-Flop Repl. ==
  S : Inport
  R : Inport  Port=2
  Logical Operator : Logic  Operator=NAND  AllPortsSameDT=off  OutDataTypeStr=boolean
  Logical Operator1 : Logic  Operator=NAND  AllPortsSameDT=off  OutDataTypeStr=boolean
  Logical Operator2 : Logic  Operator=NOT  AllPortsSameDT=off  OutDataTypeStr=boolean
  Logical Operator3 : Logic  Operator=NOT  AllPortsSameDT=off  OutDataTypeStr=boolean
  Unit Delay : UnitDelay  SampleTime=-1
  Unit Delay1 : UnitDelay  InitialCondition=1  SampleTime=-1
  Q : Outport
  !Q : Outport  Port=2
  wires:
  Logical Operator/1 -> Unit Delay1/1, !Q/1
  Logical Operator1/1 -> Unit Delay/1, Q/1
  Unit Delay/1 -> Logical Operator/1
  Unit Delay1/1 -> Logical Operator1/2
  Logical Operator2/1 -> Logical Operator1/1
  Logical Operator3/1 -> Logical Operator/2
  R/1 -> Logical Operator3/1
  S/1 -> Logical Operator2/1

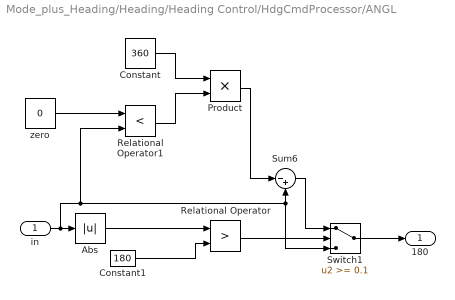
== system Mode_plus_Heading/Heading/Heading Control/HdgCmdProcessor/ANGL ==
  in : Inport  RequirementInfo={} %GIDa_3a76bb2a_5bc7_48b6_8244_4e57da04e521
  Abs : Abs
  Constant : Constant  Value=360
  Constant1 : Constant  RequirementInfo={} %GIDa_bdda2236_be0d_47e1_841c_334774b860f3  Value=180
  Product : Product  RndMeth=Zero
  Relational Operator : RelationalOperator  RequirementInfo={} %GIDa_ac754854_a082_4b35_a235_495be4fdf847  Operator=>
  Relational Operator1 : RelationalOperator  Operator=<  OutDataTypeStr=boolean
  Sum6 : Sum  RequirementInfo={} %GIDa_88f8baa6_1a02_4b52_b8c6_751e47573c97  Inputs=|-+  SaturateOnIntegerOverflow=on
  Switch1 : Switch  RequirementInfo={} %GIDa_790f289a_73f1_493b_95ff_53a70649d439  Threshold=0.1  SaturateOnIntegerOverflow=on
  zero : Constant  Value=0
  180 : Outport  RequirementInfo={} %GIDa_eab4be06_8783_4765_b34a_727109de5d2d
  wires:
  Abs/1 -> Relational Operator/1
  in/1 -> Abs/1, Switch1/3, Sum6/2, Relational Operator1/2
  Switch1/1 -> 180/1
  Product/1 -> Sum6/1
  Sum6/1 -> Switch1/1
  Relational Operator/1 -> Switch1/2
  Constant1/1 -> Relational Operator/2
  zero/1 -> Relational Operator1/1
  Constant/1 -> Product/1
  Relational Operator1/1 -> Product/2

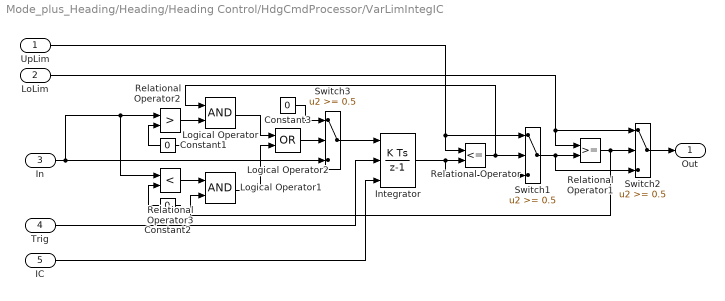
== system Mode_plus_Heading/Heading/Heading Control/HdgCmdProcessor/VarLimIntegIC ==
  UpLim : Inport  RequirementInfo={} %GIDa_65bd53f6_eca2_4cfb_b78a_b5a9cfcb0b0e
  LoLim : Inport  RequirementInfo={} %GIDa_64d96010_0a80_4501_87a7_c1c690c51c3b  Port=2
  In : Inport  RequirementInfo={} %GIDa_67b4ee9e_b607_4bf7_a18d_1fff02d99771  Port=3
  Trig : Inport  RequirementInfo={} %GIDa_d81c83b9_10e2_4876_af54_cf2467b26e7d  Port=4
  IC : Inport  RequirementInfo={} %GIDa_046bef91_7d9b_4a72_a92c_8b670143c4d8  Port=5
  Constant1 : Constant  RequirementInfo={} %GIDa_bc906e04_4b66_48c2_928b_8ec949a667c4  Value=0
  Constant2 : Constant  RequirementInfo={} %GIDa_5095fb14_b4cf_4b01_ba89_fea9fdb5b1e5  Value=0
  Constant3 : Constant  RequirementInfo={} %GIDa_ec9ff8cf_2706_4106_8ee4_987138d13e02  Value=0
  Integrator : DiscreteIntegrator  ExternalReset=level  InitialConditionSource=external  SampleTime=1.0  mask(DiscretizedDiscreteIntegrator){}
      mask init:
      | %zoh
  Logical Operator : Logic  RequirementInfo={} %GIDa_f16b325f_40c2_4832_8ad6_ad5b93c4933e  AllPortsSameDT=off
  Logical Operator1 : Logic  RequirementInfo={} %GIDa_0bd518a3_99e1_4e51_b826_8534fdb4a2a6  AllPortsSameDT=off
  Logical Operator2 : Logic  RequirementInfo={} %GIDa_5bdd1202_43af_46a7_8db1_107f29592728  Operator=OR  AllPortsSameDT=off
  Relational Operator : RelationalOperator  RequirementInfo={} %GIDa_8312b828_aec6_4750_b0fb_7f05db968a27  Operator=<=
  Relational Operator1 : RelationalOperator  RequirementInfo={} %GIDa_01147a4c_0ce6_4f26_b175_38a0dc894f0d
  Relational Operator2 : RelationalOperator  RequirementInfo={} %GIDa_6b510aba_fd31_4636_b312_1c26e54ed107  Operator=>
  Relational Operator3 : RelationalOperator  RequirementInfo={} %GIDa_62b984e9_44bd_4b8e_8413_f690aaeff84d  Operator=<
  Switch1 : Switch  RequirementInfo={} %GIDa_573e9a84_9a6f_426c_b5c1_7b08024602c8  Threshold=0.5  SaturateOnIntegerOverflow=on  InputSameDT=on
  Switch2 : Switch  RequirementInfo={} %GIDa_3ec60d4f_698b_43c3_92ce_d4e52b98cafb  Threshold=0.5  SaturateOnIntegerOverflow=on  InputSameDT=on
  Switch3 : Switch  RequirementInfo={} %GIDa_4cd76f38_5767_410b_b86a_fa3dec10e814  Threshold=0.5  SaturateOnIntegerOverflow=on  InputSameDT=on
  Out : Outport  RequirementInfo={} %GIDa_b0fbff8c_5a81_4ffb_8c3c_e4f79b7fff81
  wires:
  Relational Operator1/1 -> Logical Operator1/2, Switch2/2
  Switch1/1 -> Switch2/3, Relational Operator1/2
  LoLim/1 -> Relational Operator1/1, Switch2/1
  IC/1 -> Integrator/3
  Trig/1 -> Integrator/2
  Constant2/1 -> Relational Operator3/2
  Relational Operator3/1 -> Logical Operator1/1
  Logical Operator1/1 -> Logical Operator2/2
  Logical Operator/1 -> Logical Operator2/1
  Logical Operator2/1 -> Switch3/2
  Relational Operator2/1 -> Logical Operator/2
  Constant1/1 -> Relational Operator2/2
  In/1 -> Switch3/3, Relational Operator3/1, Relational Operator2/1
  Constant3/1 -> Switch3/1
  Switch3/1 -> Integrator/1
  Relational Operator/1 -> Logical Operator/1, Switch1/2
  Switch2/1 -> Out/1
  UpLim/1 -> Switch1/1, Relational Operator/1
  Integrator/1 -> Relational Operator/2, Switch1/3

== system Mode_plus_Heading/Heading/Roll InnerLoop/Kcas_pp/Interpolate1 ==
  InportIn : Inport
  InportIdx1 : Inport  Port=2
  InportIdx2 : Inport  Port=3
  InportData1 : Inport  Port=4
  InportData2 : Inport  Port=5
  Interpolate : Product  Inputs=*/*  SaturateOnIntegerOverflow=on  RndMeth=Zero  InputSameDT=on  OutDataTypeStr=Inherit: Same as first input
  Sum1 : Sum  Inputs=+-  SaturateOnIntegerOverflow=on  InputSameDT=on  OutDataTypeStr=Inherit: Same as first input
  Sum2 : Sum  Inputs=-+  SaturateOnIntegerOverflow=on  InputSameDT=on  OutDataTypeStr=Inherit: Same as first input
  Sum3 : Sum  Inputs=-+  SaturateOnIntegerOverflow=on  InputSameDT=on  OutDataTypeStr=Inherit: Same as first input
  Sum4 : Sum  SaturateOnIntegerOverflow=on  InputSameDT=on  OutDataTypeStr=Inherit: Same as first input
  Out : Outport
  wires:
  InportIn/1 -> Sum1/1
  InportIdx1/1 -> Sum1/2, Sum2/1
  InportIdx2/1 -> Sum2/2
  InportData1/1 -> Sum3/1, Sum4/2
  InportData2/1 -> Sum3/2
  Sum1/1 -> Interpolate/1
  Sum2/1 -> Interpolate/2
  Sum3/1 -> Interpolate/3
  Interpolate/1 -> Sum4/1
  Sum4/1 -> Out/1

== system Mode_plus_Heading/Heading/Roll InnerLoop/Kcas_pp/Interpolate2 ==
  InportIn : Inport
  InportIdx1 : Inport  Port=2
  InportIdx2 : Inport  Port=3
  InportData1 : Inport  Port=4
  InportData2 : Inport  Port=5
  Interpolate : Product  Inputs=*/*  SaturateOnIntegerOverflow=on  RndMeth=Zero  InputSameDT=on  OutDataTypeStr=Inherit: Same as first input
  Sum1 : Sum  Inputs=+-  SaturateOnIntegerOverflow=on  InputSameDT=on  OutDataTypeStr=Inherit: Same as first input
  Sum2 : Sum  Inputs=-+  SaturateOnIntegerOverflow=on  InputSameDT=on  OutDataTypeStr=Inherit: Same as first input
  Sum3 : Sum  Inputs=-+  SaturateOnIntegerOverflow=on  InputSameDT=on  OutDataTypeStr=Inherit: Same as first input
  Sum4 : Sum  SaturateOnIntegerOverflow=on  InputSameDT=on  OutDataTypeStr=Inherit: Same as first input
  Out : Outport
  wires:
  InportIn/1 -> Sum1/1
  InportIdx1/1 -> Sum1/2, Sum2/1
  InportIdx2/1 -> Sum2/2
  InportData1/1 -> Sum3/1, Sum4/2
  InportData2/1 -> Sum3/2
  Sum1/1 -> Interpolate/1
  Sum2/1 -> Interpolate/2
  Sum3/1 -> Interpolate/3
  Interpolate/1 -> Sum4/1
  Sum4/1 -> Out/1

== system Mode_plus_Heading/Heading/Roll InnerLoop/Kcas_pp/Interpolate3 ==
  InportIn : Inport
  InportIdx1 : Inport  Port=2
  InportIdx2 : Inport  Port=3
  InportData1 : Inport  Port=4
  InportData2 : Inport  Port=5
  Interpolate : Product  Inputs=*/*  SaturateOnIntegerOverflow=on  RndMeth=Zero  InputSameDT=on  OutDataTypeStr=Inherit: Same as first input
  Sum1 : Sum  Inputs=+-  SaturateOnIntegerOverflow=on  InputSameDT=on  OutDataTypeStr=Inherit: Same as first input
  Sum2 : Sum  Inputs=-+  SaturateOnIntegerOverflow=on  InputSameDT=on  OutDataTypeStr=Inherit: Same as first input
  Sum3 : Sum  Inputs=-+  SaturateOnIntegerOverflow=on  InputSameDT=on  OutDataTypeStr=Inherit: Same as first input
  Sum4 : Sum  SaturateOnIntegerOverflow=on  InputSameDT=on  OutDataTypeStr=Inherit: Same as first input
  Out : Outport
  wires:
  InportIn/1 -> Sum1/1
  InportIdx1/1 -> Sum1/2, Sum2/1
  InportIdx2/1 -> Sum2/2
  InportData1/1 -> Sum3/1, Sum4/2
  InportData2/1 -> Sum3/2
  Sum1/1 -> Interpolate/1
  Sum2/1 -> Interpolate/2
  Sum3/1 -> Interpolate/3
  Interpolate/1 -> Sum4/1
  Sum4/1 -> Out/1
